simulink model "PMSM_3PhaseCurrent"  (R2022a)
settings: Solver=FixedStepDiscrete  StartTime=0.0  StopTime=6.28  FixedStep=0.001  RelTol=1e-3
libraries: dspsrcs4 x3, simulink x3
settings Model: Creator=A  LastModifiedBy=A

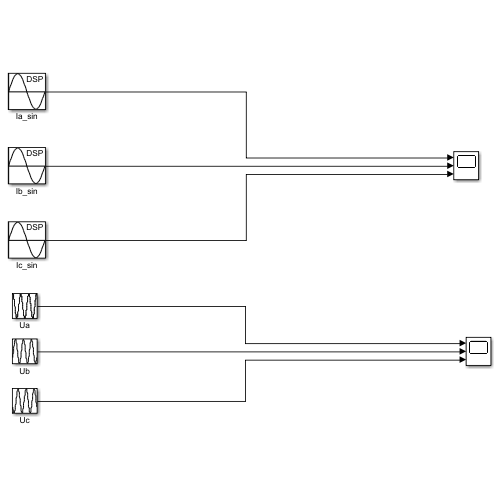
[thumbnail: Simulink's stored preview of the top-level diagram]
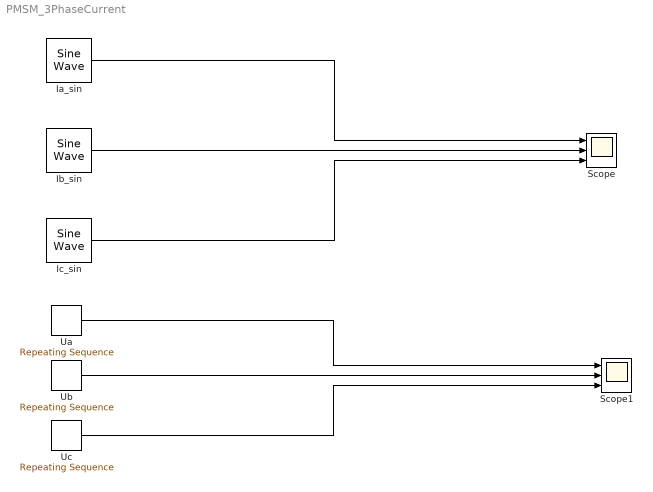
== system PMSM_3PhaseCurrent ==
  Ia_sin : dspsrcs4/Sine Wave  Amplitude=1  Frequency=1  Phase=0  SampleMode=Continuous  OutComplex=Real  CompMethod=Trigonometric fcn  TableSize=Speed  SampleTime=1/1000  SamplesPerFrame=1  ResetState=Restart at time zero  OutputFrames=off  dataType=double  wordLen=16  udDataType=sfix(16)  fracBitsMode=Best precision  numFracBits=15  OutDataTypeStr=double  LastOutDataTypeStr=double
  Ib_sin : dspsrcs4/Sine Wave  Amplitude=1  Frequency=1  Phase=2*pi/3  SampleMode=Continuous  OutComplex=Real  CompMethod=Trigonometric fcn  TableSize=Speed  SampleTime=1/1000  SamplesPerFrame=1  ResetState=Restart at time zero  OutputFrames=off  dataType=double  wordLen=16  udDataType=sfix(16)  fracBitsMode=Best precision  numFracBits=15  OutDataTypeStr=double  LastOutDataTypeStr=double
  Ic_sin : dspsrcs4/Sine Wave  Amplitude=1  Frequency=1  Phase=4*pi/3  SampleMode=Continuous  OutComplex=Real  CompMethod=Trigonometric fcn  TableSize=Speed  SampleTime=1/1000  SamplesPerFrame=1  ResetState=Restart at time zero  OutputFrames=off  dataType=double  wordLen=16  udDataType=sfix(16)  fracBitsMode=Best precision  numFracBits=15  OutDataTypeStr=double  LastOutDataTypeStr=double
  Scope : Scope  NumInputPorts=3
  Scope1 : Scope  NumInputPorts=3
  Ua : simulink/Sources/Repeating Sequence  rep_seq_t=[0:0.01:2*pi]  rep_seq_y=cos([0:0.01:2*pi])
  Ub : simulink/Sources/Repeating Sequence  rep_seq_t=[0:0.01:2*pi]  rep_seq_y=cos([0:0.01:2*pi]-2*pi/3)
  Uc : simulink/Sources/Repeating Sequence  rep_seq_t=[0:0.01:2*pi]  rep_seq_y=cos([0:0.01:2*pi]+2*pi/3)
  wires:
  Ia_sin/1 -> Scope/1
  Ib_sin/1 -> Scope/2
  Ic_sin/1 -> Scope/3
  Ua/1 -> Scope1/1
  Ub/1 -> Scope1/2
  Uc/1 -> Scope1/3
